simulink model "aeroblk_indicated"  (Simulink 6.0)
settings: Solver=FixedStepDiscrete  StartTime=0.0  StopTime=10.0  RelTol=1e-3
PreLoadFcn:
  | aeroblk_aircaldata
values from neighbouring files (symbols this model uses):
  flaps0CAS = [43 51 59 68 77 87 98 108 118 129 140]    [aeroblk_aircaldata.m]
  flaps10CAS = [42 50 60 69 78 82]    [aeroblk_aircaldata.m]
  flaps40CAS = [40 50 61 72 83 89]    [aeroblk_aircaldata.m]
libraries: simulink x3, aerolibatmos2 x1, aerolibasang x1
CloseFcn:
  | clear flaps0CAS flaps0IAS flaps10CAS flaps40CAS flaps10n40IAS
settings Model: Creator=The MathWorks Inc.  LastModifiedBy=batserve  ExtModeAutoUpdateStatusClock=off
settings DataIOCC: SaveOutput=off  SaveTime=off  SignalLoggingName=sigsOut
settings OptimizationCC: InlineParams=on
settings DebuggingCC: CheckExecutionContextPreStartOutputMsg=on  CheckExecutionContextRuntimeOutputMsg=on  SolverPrmCheckMsg=none
settings HardwareCC: TargetUnknown=on
settings RTWCC: GenCodeOnly=on

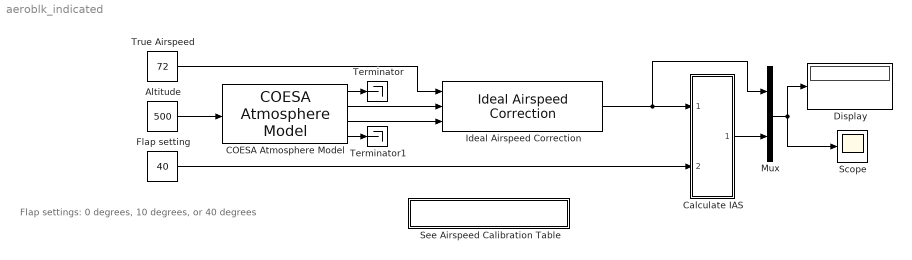
== system aeroblk_indicated ==
  note: Flap settings:
      |   0 degrees,
      | 10 degrees, or
      | 40 degrees
  Altitude : Constant  Value=500
  COESA Atmosphere Model : aerolibatmos2/COESA Atmosphere Model  units=English (Velocity in kts)  spec=1976 COESA-extended U.S. Standard Atmosphere  model=Profile  profile_var=High temperature  profile_percent=1%  profile_alt=5 km (16404 ft)  envelope_var=High temperature  envelope_percent=1%  action=Warning
  Calculate IAS : Subsystem  PropExecContextAcrossSSBoundary=on
  Display : Display
  Flap setting : Constant  Value=40
  Ideal Airspeed Correction : aerolibasang/Ideal Airspeed Correction  units=English (Velocity in kts)  vel_in=TAS  vel_out_tas=CAS  vel_out_eas=TAS  vel_out_cas=EAS  action=Error
  Mux : Mux  Inputs=2
  Scope : Scope
      settings: TimeRange=10  YMin=69.5  YMax=71.5
  See Airspeed Calibration Table : Subsystem  PropExecContextAcrossSSBoundary=on
      settings: OpenFcn=open('aeroblk_aircaldata.m');
      mask Display: disp('Cessna 150M Commuter');
  Terminator : Terminator
  Terminator1 : Terminator
  True Airspeed : Constant  Value=72
  wires:
  True Airspeed/1 -> Ideal Airspeed Correction/1
  Ideal Airspeed Correction/1 -> Calculate IAS/1(CAS), Mux/1
  COESA Atmosphere Model/3 -> Ideal Airspeed Correction/3
  COESA Atmosphere Model/2 -> Ideal Airspeed Correction/2
  COESA Atmosphere Model/4 -> Terminator1/1
  COESA Atmosphere Model/1 -> Terminator/1
  Altitude/1 -> COESA Atmosphere Model/1
  Flap setting/1 -> Calculate IAS/2(Flap)
  Calculate IAS/1(IAS) -> Mux/2
  Mux/1 -> Display/1, Scope/1

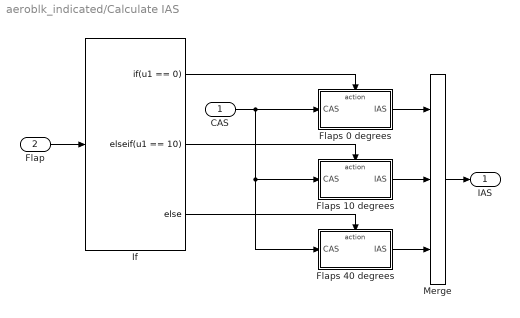
== system aeroblk_indicated/Calculate IAS ==
  CAS : Inport  Port=1  LatchInput=off
  Flap : Inport  Port=2  LatchInput=off
  Flaps 0 degrees : Subsystem  TreatAsAtomicUnit=on  PropExecContextAcrossSSBoundary=on
  Flaps 10 degrees : Subsystem  TreatAsAtomicUnit=on  PropExecContextAcrossSSBoundary=on
  Flaps 40 degrees : Subsystem  TreatAsAtomicUnit=on  PropExecContextAcrossSSBoundary=on
  If : If  IfExpression=u1 == 0  ElseIfExpressions=u1 == 10
  Merge : Merge  Inputs=3
  IAS : Outport
  wires:
  If/1 -> Flaps 0 degrees/Action
  If/2 -> Flaps 10 degrees/Action
  If/3 -> Flaps 40 degrees/Action
  CAS/1 -> Flaps 0 degrees/1(CAS), Flaps 10 degrees/1(CAS), Flaps 40 degrees/1(CAS)
  Flaps 0 degrees/1(IAS) -> Merge/1
  Flap/1 -> If/1
  Flaps 10 degrees/1(IAS) -> Merge/2
  Flaps 40 degrees/1(IAS) -> Merge/3
  Merge/1 -> IAS/1

== system aeroblk_indicated/See Airspeed Calibration Table ==

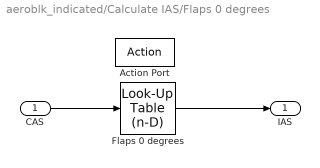
== system aeroblk_indicated/Calculate IAS/Flaps 0 degrees ==
  CAS : Inport  Port=1  LatchInput=off
  Action Port : ActionPort  ActionType=then
  Flaps 0 degrees : simulink/Look-Up Tables/Look-Up Table (n-D)  numDimsPopupSelect=1  bp1=flaps0CAS  bp2=[10,22,31]  bp3=[1:3]  bp4=[1:3]  bpcell={ [1:3], [1:3] }  explicitNumDims=2  searchMode=Binary Search  cacheBpFlag=on  vectorInputFlag=on  tableData=flaps0IAS  interpMethod=Linear  extrapMethod=None - Clip  rangeErrorMode=Warning
  IAS : Outport
  wires:
  CAS/1 -> Flaps 0 degrees/1
  Flaps 0 degrees/1 -> IAS/1

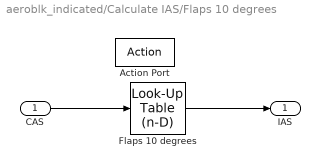
== system aeroblk_indicated/Calculate IAS/Flaps 10 degrees ==
  CAS : Inport  Port=1  LatchInput=off
  Action Port : ActionPort  ActionType=elseif
  Flaps 10 degrees : simulink/Look-Up Tables/Look-Up Table (n-D)  numDimsPopupSelect=1  bp1=flaps10CAS  bp2=[10,22,31]  bp3=[1:3]  bp4=[1:3]  bpcell={ [1:3], [1:3] }  explicitNumDims=2  searchMode=Binary Search  cacheBpFlag=on  vectorInputFlag=on  tableData=flaps10n40IAS  interpMethod=Linear  extrapMethod=None - Clip  rangeErrorMode=Warning
  IAS : Outport
  wires:
  CAS/1 -> Flaps 10 degrees/1
  Flaps 10 degrees/1 -> IAS/1

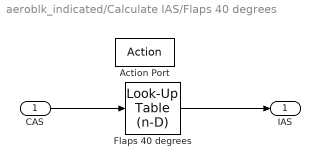
== system aeroblk_indicated/Calculate IAS/Flaps 40 degrees ==
  CAS : Inport  Port=1  LatchInput=off
  Action Port : ActionPort  ActionType=else
  Flaps 40 degrees : simulink/Look-Up Tables/Look-Up Table (n-D)  numDimsPopupSelect=1  bp1=flaps40CAS  bp2=[10,22,31]  bp3=[1:3]  bp4=[1:3]  bpcell={ [1:3], [1:3] }  explicitNumDims=2  searchMode=Binary Search  cacheBpFlag=on  vectorInputFlag=on  tableData=flaps10n40IAS  interpMethod=Linear  extrapMethod=None - Clip  rangeErrorMode=Warning
  IAS : Outport
  wires:
  CAS/1 -> Flaps 40 degrees/1
  Flaps 40 degrees/1 -> IAS/1
